simulink model "test_detection_front_national"  (R2014a)
settings: Solver=ode45  StartTime=0.0  StopTime=10.0  RelTol=1e-3
libraries: simulink x1
settings Model: Creator=elkhadiy  LastModifiedBy=elkhadiy

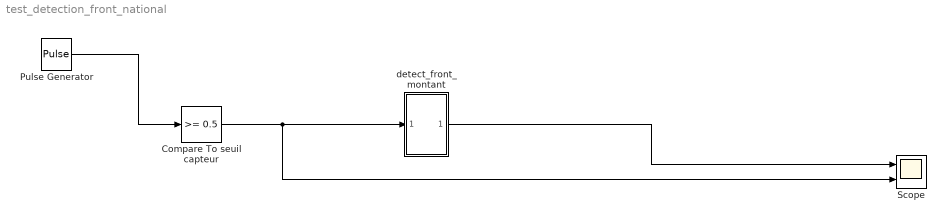
== system test_detection_front_national ==
  Compare To seuil capteur : simulink/Logic and Bit Operations/Compare To Constant  relop=>=  const=0.5  OutDataTypeStr=boolean
  Pulse Generator : DiscretePulseGenerator  PulseType=Time based  Period=3  PulseWidth=50
  Scope : Scope  NumInputPorts=2
      settings: YMin=-5~-5  YMax=5~5
  detect_front_montant : Subsystem
  wires:
  Pulse Generator/1 -> Compare To seuil capteur/1
  Compare To seuil capteur/1 -> Scope/2, detect_front_montant/1(In1)
  detect_front_montant/1(Out1) -> Scope/1

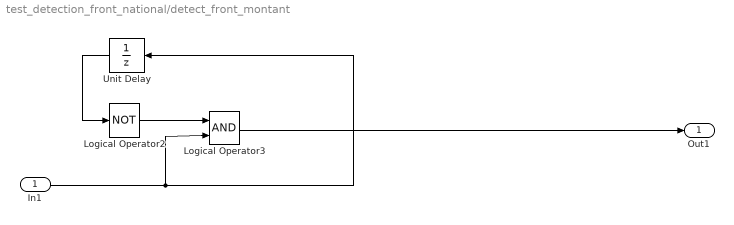
== system test_detection_front_national/detect_front_montant ==
  In1 : Inport
  Logical Operator2 : Logic  Operator=NOT  AllPortsSameDT=off  OutDataTypeStr=boolean
  Logical Operator3 : Logic  AllPortsSameDT=off  OutDataTypeStr=boolean
  Unit Delay : UnitDelay  SampleTime=-1
  Out1 : Outport
  wires:
  In1/1 -> Unit Delay/1, Logical Operator3/2
  Logical Operator2/1 -> Logical Operator3/1
  Unit Delay/1 -> Logical Operator2/1
  Logical Operator3/1 -> Out1/1
